simulink model "System"  (R2019b)
settings: Solver=VariableStepAuto  StartTime=0.0  StopTime=10.0  RelTol=1e-3
PreLoadFcn:
  | load AllBuses
settings Model: Creator=Lenovo  LastModifiedBy=Lenovo
settings OptimizationCC: DefaultParameterBehavior=Inlined

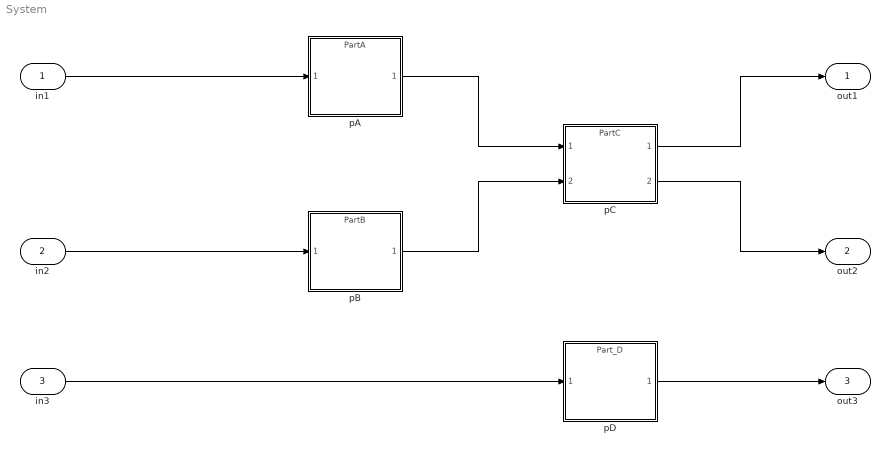
== system System ==
  in1 : Inport  OutDataTypeStr=Bus: Bus_1  BusOutputAsStruct=on
  in2 : Inport  Port=2  OutDataTypeStr=int32
  in3 : Inport  Port=3  OutDataTypeStr=Bus: Bus_2  BusOutputAsStruct=on
  pA : ModelReference  ModelNameDialog=PartA  SimulationMode=Normal  ModelReferenceVersion=1.1
  pB : ModelReference  ModelNameDialog=PartB  SimulationMode=Normal  ModelReferenceVersion=1.1
  pC : ModelReference  ModelNameDialog=PartC  SimulationMode=Normal  ModelReferenceVersion=1.1
  pD : ModelReference  ModelNameDialog=Part_D  SimulationMode=Normal  ModelReferenceVersion=1.1
  out1 : Outport  OutDataTypeStr=double
  out2 : Outport  Port=2  OutDataTypeStr=boolean
  out3 : Outport  Port=3  OutDataTypeStr=Bus: Bus_3  BusOutputAsStruct=on
  wires:
  in1/1 -> pA/1
  in2/1 -> pB/1
  pD/1 -> out3/1
  pA/1 -> pC/1
  pB/1 -> pC/2
  pC/1 -> out1/1
  pC/2 -> out2/1
  in3/1 -> pD/1
